simulink model "psm_svpwm_nonlinear_ctrl"  (R2026a)
settings: Solver=ode23tb  StopTime=simlength  FixedStep=tc  MaxStep=tc
values from neighbouring files (symbols this model uses):
  CTRPIFF_CLIP_RELEASE = 0.001    [init_model.m]
  dead_time_INV = 3e-6    (= 3e-06)    [init_model.m]
  emf_fb_p = 0.2    [init_model.m]
  emf_fb_p_ccaller_1 = emf_fb_p    (= 0.2)    [init_model.m]
  emf_fb_p_ccaller_2 = emf_fb_p    (= 0.2)    [init_model.m]
  emf_p = emf_fb_p*4/10    (= 0.08)    [init_model.m]
  emf_p_ccaller_1 = emf_fb_p_ccaller_1*4/10    (= 0.08)    [init_model.m]
  emf_p_ccaller_2 = emf_fb_p_ccaller_2*4/10    (= 0.08)    [init_model.m]
  fPWM_INV = fPWM_AFE    (= 5000)    [init_model.m]
  g0_10Hz = fcut_10Hz_flt * ts_afe * 2*pi    (= 0.0125663706144)    [init_model.m]
  g0_1Hz = fcut_1Hz_flt * ts_afe * 2*pi    (= 0.00125663706144)    [init_model.m]
  g1_10Hz = 1 - g0_10Hz    (= 0.987433629386)    [init_model.m]
  g1_1Hz = 1 - g0_1Hz    (= 0.998743362939)    [init_model.m]
  id_lim = 0.35    [init_model.m]
  inv_m_scale = motorc_m_scale    [init_model.m]
  iq_lim = 1.4    [init_model.m]
  kg = Kobs(1)    [init_model.m]
  ki_align = 0.1    [init_model.m]
  ki_i = 18    [init_model.m]
  ki_w = 8    [init_model.m]
  kp_align = 0.6    [init_model.m]
  kp_i = 0.25    [init_model.m]
  kp_w = 2    [init_model.m]
  kw = Kobs(2)    [init_model.m]
  lim_down_align = -0.2    [init_model.m]
  lim_up_align = 0.2    [init_model.m]
  number_of_modules = 1    [init_model.m]
  omega_m_sim = omega_m_bez    [init_model.m]
  simlength = 2    [init_model.m]
  tc = ts_afe/100    (= 2e-06)    [init_model.m]
  time_gain_afe_module_1 = 1.0    (= 1)    [init_model.m]
  time_gain_inv_module_2 = 1.0    (= 1)    [init_model.m]
  time_start_motor_control = 0.025    [init_model.m]
  ts_inv = 1/fPWM_INV    (= 0.0002)    [init_model.m]
undefined symbols (not defined in the file or in its folder): ibez, La, Lb, Ld_norm, Lq_norm, Ls_norm, magnitude, omega_bez, omega_m_bez, psi_bez, psi_m, psi_m_norm, rpm_base, rpm_bez, Rs, Rs_norm, tau_bez, torque_base, ubez
libraries: fl_lib x24, nesl_utility x11, cstblocks_lti x2, single_phase_pwm_modulator x1, pi_ctrl x1, threephase_inductor_lib x1, simple_flexible_shaft x1, permanent_magnet_synchronous_machine x1
(part 3 of 3)

== system psm_svpwm_nonlinear_ctrl/inv_psm_mod1/inverter_ctrl/inverter_control/current_ctrl/current_ctrl/dq_pi_with_vector_antiwindup mod1/dq_vector_pi ==
  id : Inport
  id_ref : Inport  Port=2
  iq : Inport  Port=3
  iq_ref : Inport  Port=4
  Sum1 : Sum  Inputs=|-+
  Sum2 : Sum  Inputs=|-+
  bounder1 : Subsystem
  bounder2 : Subsystem
  pi_d : Subsystem
  pi_q : Subsystem
  switch : Subsystem
  vector lenght : Subsystem
  md_sat : Outport
  mq_sat : Outport  Port=2
  wires:
  bounder2/2(clip) -> switch/2(clip 2)
  vector lenght/2(m) -> bounder1/3(m), bounder2/1(m)
  Sum2/1 -> pi_q/1(iq_tilde)
  pi_d/1(ud_out) -> vector lenght/1(md), bounder1/1(md)
  pi_q/1(Vqs_out) -> bounder2/3(mq), vector lenght/2(mq)
  vector lenght/1(m_1) -> bounder1/2(m_1), bounder2/2(m_1)
  switch/1(clip) -> pi_q/2(clip), pi_d/2(clip)
  iq/1 -> Sum2/1
  Sum1/1 -> pi_d/1(id_tilde)
  bounder1/2(clip) -> switch/1(clip 1)
  id/1 -> Sum1/1
  bounder1/1(md_sat) -> md_sat/1
  bounder2/1(mq_sat) -> mq_sat/1
  id_ref/1 -> Sum1/2
  iq_ref/1 -> Sum2/2

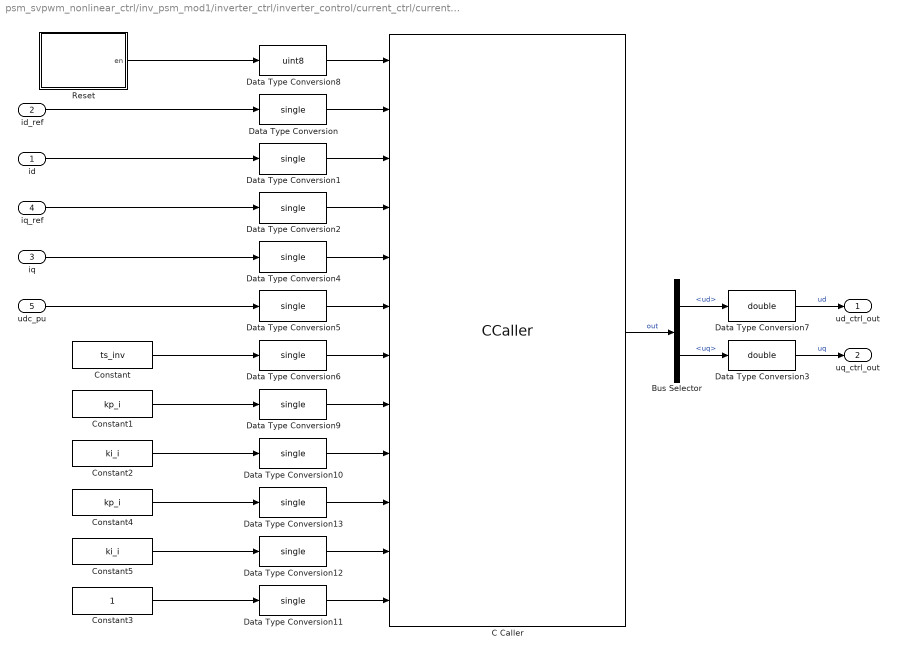
== system psm_svpwm_nonlinear_ctrl/inv_psm_mod1/inverter_ctrl/inverter_control/current_ctrl/current_ctrl/dq_pi_with_vector_antiwindup mod1/dq_vector_pi_ccaller ==
  id : Inport
  id_ref : Inport  Port=2
  iq : Inport  Port=3
  iq_ref : Inport  Port=4
  udc_pu : Inport  Port=5
  Bus Selector : BusSelector  OutputSignals=ud,uq
  C Caller : CCaller  FunctionName=dqvector_pi_process_simulink  PortSpecificationStruct="%)30     .    ,!8   8    (     @         %    \"     T    !     0         %  0 \"0    $    _    07)G3F%M90  4&]R=$YA;64 4V-O<&4     26YD97@     5'EP90      4VEZ90      27-';&]B86P   X    P    !@    @    $          4    (     0    ,    !         !   P!O=70 #@   #     &    \"     0         !0    @    !     P    $         $  # &]U=  .    .     8    (    !          %    \"     $    &     0         0   ...(+7280 chars)"
  Constant : Constant  Value=ts_inv
  Constant1 : Constant  Value=kp_i
  Constant2 : Constant  Value=ki_i
  Constant3 : Constant
  Constant4 : Constant  Value=kp_i
  Constant5 : Constant  Value=ki_i
  Data Type Conversion{,1..2,4..6,9..13} (11 alike) : DataTypeConversion  OutDataTypeStr=single  SaturateOnIntegerOverflow=off  RndMeth=Floor
  Data Type Conversion3 : DataTypeConversion  OutDataTypeStr=double  SaturateOnIntegerOverflow=off  RndMeth=Floor
  Data Type Conversion7 : DataTypeConversion  OutDataTypeStr=double  SaturateOnIntegerOverflow=off  RndMeth=Floor
  Data Type Conversion8 : DataTypeConversion  OutDataTypeStr=uint8  SaturateOnIntegerOverflow=off  RndMeth=Floor
  Reset : Subsystem
  ud_ctrl_out : Outport
  uq_ctrl_out : Outport  Port=2
  wires:
  Data Type Conversion5/1 -> C Caller/6
  Data Type Conversion/1 -> C Caller/2
  C Caller/1 -> Bus Selector/1  "out"
  Data Type Conversion1/1 -> C Caller/3
  Data Type Conversion4/1 -> C Caller/5
  Data Type Conversion2/1 -> C Caller/4
  Data Type Conversion6/1 -> C Caller/7
  Bus Selector/2 -> Data Type Conversion3/1  "<uq>"
  Bus Selector/1 -> Data Type Conversion7/1  "<ud>"
  Data Type Conversion7/1 -> ud_ctrl_out/1  "ud"
  Data Type Conversion3/1 -> uq_ctrl_out/1  "uq"
  Data Type Conversion8/1 -> C Caller/1
  Data Type Conversion9/1 -> C Caller/8
  Data Type Conversion10/1 -> C Caller/9
  Data Type Conversion11/1 -> C Caller/12
  Data Type Conversion13/1 -> C Caller/10
  Data Type Conversion12/1 -> C Caller/11
  Constant3/1 -> Data Type Conversion11/1
  Constant5/1 -> Data Type Conversion12/1
  Constant4/1 -> Data Type Conversion13/1
  Constant2/1 -> Data Type Conversion10/1
  Constant1/1 -> Data Type Conversion9/1
  Constant/1 -> Data Type Conversion6/1
  udc_pu/1 -> Data Type Conversion5/1
  iq/1 -> Data Type Conversion4/1
  iq_ref/1 -> Data Type Conversion2/1
  Reset/1(en) -> Data Type Conversion8/1
  id_ref/1 -> Data Type Conversion/1
  id/1 -> Data Type Conversion1/1

== system psm_svpwm_nonlinear_ctrl/inv_psm_mod1/inverter_ctrl/inverter_control/current_ctrl/bemf_observer/nonlinear_observer/phase_lock_loop/theta_bemf_hat ==
  psi_sd_hat : Inport
  psi_sq_hat : Inport  Port=2
  omega_hat : Inport  Port=3
  Constant1 : Constant  Value=0
  Constant2 : Constant  Value=0
  Gain : Gain  Gain=-1
  Gain1 : Gain  Commented=on  Gain=-1
  Sum : Sum  Inputs=|++
  Trigonometric Function : Trigonometry  Operator=atan2  OutputSignalType=real
  alignment : Scope  NumInputPorts=2
      settings: ActiveDisplayYMinimum=-1.4296113114155271  ActiveDisplayYMaximum=2.2501138881400213  DataLoggingVariableName=ScopeData5
  damped_integral : Subsystem  Commented=on  mask{omega_bez_m=omega_bez, damping_m=0.01, ts_m=ts_inv}
      mask prompts: omega_bez_m "omega_bez"; damping_m "damping"; ts_m "ts"
  damped_integral_with_mod : Subsystem  mask{omega_bez_m=omega_bez, damping_m=0, ts_m=ts_inv}
      mask prompts: omega_bez_m "omega_bez"; damping_m "damping"; ts_m "ts"
  double_integrator_observer : Subsystem  Commented=on
  pi_ctrl : pi_ctrl/pi_ctrl  kp=1  ki=1  ts=ts_inv  lim_up=2  lim_down=-2
  omega_z : Outport  VectorParamsAs1DForOutWhenUnconnected=off
  theta_z : Outport  Port=2  VectorParamsAs1DForOutWhenUnconnected=off
  wires:
  Constant1/1 -> pi_ctrl/1
  Constant2/1 -> pi_ctrl/3
  psi_sq_hat/1 -> Trigonometric Function/1
  Gain1/1 -> double_integrator_observer/1(theta)
  damped_integral_with_mod/1(out) -> theta_z/1
  Sum/1 -> damped_integral_with_mod/1(in), alignment/2, omega_z/1
  psi_sd_hat/1 -> Trigonometric Function/2
  Gain/1 -> pi_ctrl/2
  pi_ctrl/1 -> Sum/1
  omega_hat/1 -> Sum/2
  Trigonometric Function/1 -> Gain/1, alignment/1

== system psm_svpwm_nonlinear_ctrl/inv_psm_mod1/inverter_ctrl/inverter_control/current_ctrl/bemf_observer/nonlinear_observer/psi_dq_hat/psi_d_hat ==
  Gain1 : Gain  Gain=Rs_norm
  Gain3 : Gain  Gain=emf_p
  Gain4 : Gain  Gain=omega_bez
  Gain7 : Gain  Gain=ts_inv
  Product : Product
  Sum : Sum  Inputs=|+-
  Sum2 : Sum  Inputs=++-  SaturateOnIntegerOverflow=on
  Sum3 : Sum  Inputs=|++
  Unit Delay1 : UnitDelay  SampleTime=-1
  tag scope: psi_d_hat_simulink=scoped
  wires:
  Unit Delay1/1 -> Sum3/2, Gain3/1
  Sum2/1 -> Gain4/1
  Gain7/1 -> Sum3/1
  [id_pu_m] -> Gain1/1
  [ud_pu_m] -> Sum/1
  Sum3/1 -> Unit Delay1/1, [psi_d_hat_simulink]
  Gain3/1 -> Sum2/3
  Gain4/1 -> Gain7/1
  Gain1/1 -> Sum/2
  Sum/1 -> Sum2/2
  [omega_z_pu_hat] -> Product/2
  Product/1 -> Sum2/1
  [psi_q_hat_simulink] -> Product/1

== system psm_svpwm_nonlinear_ctrl/inv_psm_mod1/inverter_ctrl/inverter_control/current_ctrl/bemf_observer/nonlinear_observer/psi_dq_hat/psi_q_hat ==
  Gain : Gain  Gain=-1
  Gain1 : Gain  Gain=Rs_norm
  Gain3 : Gain  Gain=emf_p
  Gain4 : Gain  Gain=omega_bez
  Gain7 : Gain  Gain=ts_inv
  Product : Product
  Sum : Sum  Inputs=|+-
  Sum2 : Sum  Inputs=++-  SaturateOnIntegerOverflow=on
  Sum3 : Sum  Inputs=|++
  Unit Delay1 : UnitDelay  SampleTime=-1
  tag scope: psi_q_hat_simulink=scoped
  wires:
  [omega_z_pu_hat] -> Product/2
  Sum/1 -> Sum2/2
  Gain1/1 -> Sum/2
  Gain4/1 -> Gain7/1
  Gain3/1 -> Sum2/3
  Sum3/1 -> [psi_q_hat_simulink], Unit Delay1/1
  [uq_pu_m] -> Sum/1
  [iq_pu_m] -> Gain1/1
  Gain7/1 -> Sum3/1
  Sum2/1 -> Gain4/1
  Unit Delay1/1 -> Sum3/2, Gain3/1
  Product/1 -> Gain/1
  Gain/1 -> Sum2/1
  [psi_d_hat_simulink] -> Product/1

== system psm_svpwm_nonlinear_ctrl/inv_psm_mod1/inverter_ctrl/inverter_control/current_ctrl/current_ctrl/dq_pi_with_vector_antiwindup mod1/dq_vector_pi/bounder1 ==
  md : Inport
  m_1 : Inport  Port=2
  m : Inport  Port=3
  Constant : Constant
  Constant1 : Constant  Value=0
  Divide : Product
  Switch : Switch  Threshold=1  SaturateOnIntegerOverflow=off  InputSameDT=off
  Switch1 : Switch  Threshold=1  SaturateOnIntegerOverflow=off  InputSameDT=off
  md_sat : Outport  VectorParamsAs1DForOutWhenUnconnected=off
  clip : Outport  Port=2  VectorParamsAs1DForOutWhenUnconnected=off
  wires:
  md/1 -> Switch1/3, Divide/2
  m_1/1 -> Divide/1
  Divide/1 -> Switch1/1
  Switch1/1 -> md_sat/1
  Switch/1 -> clip/1
  m/1 -> Switch/2, Switch1/2
  Constant/1 -> Switch/1
  Constant1/1 -> Switch/3

== system psm_svpwm_nonlinear_ctrl/inv_psm_mod1/inverter_ctrl/inverter_control/current_ctrl/current_ctrl/dq_pi_with_vector_antiwindup mod1/dq_vector_pi/bounder2 ==
  m : Inport
  m_1 : Inport  Port=2
  mq : Inport  Port=3
  Constant : Constant
  Constant1 : Constant  Value=0
  Divide : Product
  Switch : Switch  Threshold=1  SaturateOnIntegerOverflow=off  InputSameDT=off
  Switch1 : Switch  Threshold=1  SaturateOnIntegerOverflow=off  InputSameDT=off
  mq_sat : Outport  VectorParamsAs1DForOutWhenUnconnected=off
  clip : Outport  Port=2  VectorParamsAs1DForOutWhenUnconnected=off
  wires:
  Constant1/1 -> Switch/3
  Constant/1 -> Switch/1
  m/1 -> Switch1/2, Switch/2
  Switch/1 -> clip/1
  Switch1/1 -> mq_sat/1
  Divide/1 -> Switch1/1
  m_1/1 -> Divide/1
  mq/1 -> Divide/2, Switch1/3

== system psm_svpwm_nonlinear_ctrl/inv_psm_mod1/inverter_ctrl/inverter_control/current_ctrl/current_ctrl/dq_pi_with_vector_antiwindup mod1/dq_vector_pi/pi_d ==
  id_tilde : Inport
  clip : Inport  Port=2
  1/Ti : Gain  Gain=kp_i  SaturateOnIntegerOverflow=on  OutDataTypeStr=Inherit: Same as input  ParamDataTypeStr=Inherit: Same as input
  Constant : Constant  Value=0
  Sum2 : Sum  Inputs=+-  SaturateOnIntegerOverflow=on
  Sum4 : Sum  SaturateOnIntegerOverflow=on
  Sum5 : Sum  SaturateOnIntegerOverflow=on
  Switch1 : Switch  Threshold=0.5  SaturateOnIntegerOverflow=off  InputSameDT=off
  Switch2 : Switch  Threshold=0.5  SaturateOnIntegerOverflow=off  InputSameDT=off
  Unit Delay1 : UnitDelay  SampleTime=-1
  Unit Delay2 : UnitDelay  SampleTime=-1
  kp1 : Gain  Gain=CTRPIFF_CLIP_RELEASE*ts_inv  SaturateOnIntegerOverflow=on  OutDataTypeStr=Inherit: Same as input  ParamDataTypeStr=Inherit: Same as input
  kp2 : Gain  Gain=ki_i*ts_inv  SaturateOnIntegerOverflow=on  OutDataTypeStr=Inherit: Same as input  ParamDataTypeStr=Inherit: Same as input
  ud_out : Outport  VectorParamsAs1DForOutWhenUnconnected=off
  wires:
  id_tilde/1 -> kp2/1, 1/Ti/1
  Sum5/1 -> ud_out/1
  Switch1/1 -> Unit Delay2/1
  Sum4/1 -> Sum5/2, Switch1/3
  kp1/1 -> Sum2/2
  Sum2/1 -> Switch1/1
  Unit Delay2/1 -> Sum4/2, kp1/1, Sum2/1
  1/Ti/1 -> Sum5/1
  Switch2/1 -> Sum4/1
  kp2/1 -> Switch2/3
  clip/1 -> Unit Delay1/1
  [clip] -> Switch2/2
  [clip] -> Switch1/2
  Constant/1 -> Switch2/1
  Unit Delay1/1 -> [clip]

== system psm_svpwm_nonlinear_ctrl/inv_psm_mod1/inverter_ctrl/inverter_control/current_ctrl/current_ctrl/dq_pi_with_vector_antiwindup mod1/dq_vector_pi/pi_q ==
  iq_tilde : Inport
  clip : Inport  Port=2
  1/Ti : Gain  Gain=kp_i  SaturateOnIntegerOverflow=on  OutDataTypeStr=Inherit: Same as input  ParamDataTypeStr=Inherit: Same as input
  Constant : Constant  Value=0
  Sum2 : Sum  Inputs=+-  SaturateOnIntegerOverflow=on
  Sum4 : Sum  SaturateOnIntegerOverflow=on
  Sum5 : Sum  SaturateOnIntegerOverflow=on
  Switch1 : Switch  Threshold=0.5  SaturateOnIntegerOverflow=off  InputSameDT=off
  Switch2 : Switch  Threshold=0.5  SaturateOnIntegerOverflow=off  InputSameDT=off
  Unit Delay1 : UnitDelay  SampleTime=-1
  Unit Delay2 : UnitDelay  SampleTime=-1
  kp1 : Gain  Gain=CTRPIFF_CLIP_RELEASE*ts_inv  SaturateOnIntegerOverflow=on  OutDataTypeStr=Inherit: Same as input  ParamDataTypeStr=Inherit: Same as input
  kp2 : Gain  Gain=ki_i*ts_inv  SaturateOnIntegerOverflow=on  OutDataTypeStr=Inherit: Same as input  ParamDataTypeStr=Inherit: Same as input
  Vqs_out : Outport  VectorParamsAs1DForOutWhenUnconnected=off
  wires:
  Constant/1 -> Switch2/1
  [clip] -> Switch1/2
  [clip] -> Switch2/2
  clip/1 -> Unit Delay1/1
  kp2/1 -> Switch2/3
  Switch2/1 -> Sum4/1
  1/Ti/1 -> Sum5/1
  Unit Delay2/1 -> Sum2/1, kp1/1, Sum4/2
  Sum2/1 -> Switch1/1
  kp1/1 -> Sum2/2
  Sum4/1 -> Sum5/2, Switch1/3
  Switch1/1 -> Unit Delay2/1
  iq_tilde/1 -> 1/Ti/1, kp2/1
  Unit Delay1/1 -> [clip]
  Sum5/1 -> Vqs_out/1

== system psm_svpwm_nonlinear_ctrl/inv_psm_mod1/inverter_ctrl/inverter_control/current_ctrl/current_ctrl/dq_pi_with_vector_antiwindup mod1/dq_vector_pi/switch ==
  clip 1 : Inport
  clip 2 : Inport  Port=2
  Constant4 : Constant
  Constant5 : Constant  Value=0
  Sum1 : Sum  SaturateOnIntegerOverflow=on
  Switch : Switch  Threshold=0.5  SaturateOnIntegerOverflow=off  InputSameDT=off
  clip : Outport  VectorParamsAs1DForOutWhenUnconnected=off
  wires:
  Constant5/1 -> Switch/3
  Switch/1 -> clip/1
  Constant4/1 -> Switch/1
  Sum1/1 -> Switch/2
  clip 1/1 -> Sum1/1
  clip 2/1 -> Sum1/2

== system psm_svpwm_nonlinear_ctrl/inv_psm_mod1/inverter_ctrl/inverter_control/current_ctrl/current_ctrl/dq_pi_with_vector_antiwindup mod1/dq_vector_pi/vector lenght ==
  md : Inport
  mq : Inport  Port=2
  Math Function : Math  Operator=magnitude^2  SignedPower=on
  Math Function1 : Math  Operator=magnitude^2  SignedPower=on
  Math Function2 : Math  Operator=reciprocal  SignedPower=on
  Sqrt : Sqrt
  Sum5 : Sum  SaturateOnIntegerOverflow=on
  m_1 : Outport  VectorParamsAs1DForOutWhenUnconnected=off
  m : Outport  Port=2  VectorParamsAs1DForOutWhenUnconnected=off
  wires:
  Sqrt/1 -> m/1, Math Function2/1
  mq/1 -> Math Function1/1
  Math Function1/1 -> Sum5/2
  Math Function/1 -> Sum5/1
  Sum5/1 -> Sqrt/1
  Math Function2/1 -> m_1/1
  md/1 -> Math Function/1

== system psm_svpwm_nonlinear_ctrl/inv_psm_mod1/inverter_ctrl/inverter_control/current_ctrl/current_ctrl/dq_pi_with_vector_antiwindup mod1/dq_vector_pi_ccaller/Reset ==
  Step : Step  Time=0.05  InitialValue=1  FinalValue=0
  en : Outport
  wires:
  Step/1 -> en/1

== system psm_svpwm_nonlinear_ctrl/inv_psm_mod1/inverter_ctrl/inverter_control/current_ctrl/bemf_observer/nonlinear_observer/phase_lock_loop/theta_bemf_hat/damped_integral ==
  in : Inport
  Gain3 : Gain  Gain=damping_m
  Gain4 : Gain  Gain=omega_bez_m
  Gain7 : Gain  Gain=ts_m
  Sum2 : Sum  Inputs=+-  SaturateOnIntegerOverflow=on
  Sum3 : Sum  Inputs=|++
  Unit Delay1 : UnitDelay  SampleTime=-1
  out : Outport
  wires:
  Sum2/1 -> Gain4/1
  Gain7/1 -> Sum3/1
  Sum3/1 -> Unit Delay1/1
  Unit Delay1/1 -> Gain3/1, Sum3/2, out/1
  Gain4/1 -> Gain7/1
  in/1 -> Sum2/1
  Gain3/1 -> Sum2/2

== system psm_svpwm_nonlinear_ctrl/inv_psm_mod1/inverter_ctrl/inverter_control/current_ctrl/bemf_observer/nonlinear_observer/phase_lock_loop/theta_bemf_hat/damped_integral_with_mod ==
  in : Inport
  Gain3 : Gain  Gain=damping_m
  Gain4 : Gain  Gain=omega_bez_m
  Gain7 : Gain  Gain=ts_m
  Sum2 : Sum  Inputs=+-  SaturateOnIntegerOverflow=on
  Sum3 : Sum  Inputs=|++
  Unit Delay1 : UnitDelay  SampleTime=-1
  bounder1 : MATLAB Function  TreatAsAtomicUnit=on
  out : Outport
  wires:
  Gain3/1 -> Sum2/2
  in/1 -> Sum2/1
  Gain4/1 -> Gain7/1
  Unit Delay1/1 -> bounder1/1(u)
  Sum3/1 -> Unit Delay1/1
  Gain7/1 -> Sum3/1
  Sum2/1 -> Gain4/1
  bounder1/1(y) -> out/1, Sum3/2, Gain3/1

== system psm_svpwm_nonlinear_ctrl/inv_psm_mod1/inverter_ctrl/inverter_control/current_ctrl/bemf_observer/nonlinear_observer/phase_lock_loop/theta_bemf_hat/double_integrator_observer ==
  theta : Inport
  Gain : Gain  Gain=kw
  Gain1 : Gain  Gain=kg
  Gain2 : Gain  Gain=omega_bez
  Gain3 : Gain  Gain=1/omega_bez
  Gain5 : Gain  Gain=ts_inv
  Sum : Sum  Inputs=-+|
  Sum1 : Sum  Inputs=|++
  Sum2 : Sum  Inputs=|++
  Sum8 : Sum  Inputs=++|
  Unit Delay1 : UnitDelay  InitialCondition=pi  SampleTime=-1
  Unit Delay2 : UnitDelay  SampleTime=-1
  bounder1 : MATLAB Function  TreatAsAtomicUnit=on
  bounder2 : MATLAB Function  TreatAsAtomicUnit=on
  omega_z_pu_hat : Outport  VectorParamsAs1DForOutWhenUnconnected=off
  theta_z_hat : Outport  Port=2  VectorParamsAs1DForOutWhenUnconnected=off
  wires:
  Gain1/1 -> Sum2/1
  theta/1 -> Sum/2  "theta_bemf"
  Sum8/1 -> Unit Delay1/1
  Unit Delay1/1 -> bounder2/1(u)
  Sum1/1 -> Unit Delay2/1
  Gain/1 -> Gain3/1
  Unit Delay2/1 -> omega_z_pu_hat/1, Sum1/2, Gain5/1
  Sum2/1 -> Sum8/2
  bounder2/1(y) -> Sum2/2, theta_z_hat/1, Sum/1
  bounder1/1(y) -> Gain1/1, Gain/1
  Gain2/1 -> Sum8/1
  Gain3/1 -> Sum1/1
  Gain5/1 -> Gain2/1
  Sum/1 -> bounder1/1(u)

== matlab function psm_svpwm_nonlinear_ctrl/inv_psm_mod1/inverter_ctrl/inverter_control/current_ctrl/current_transformation/alphabeta2dq ==
  data: alpha input; d output; beta input; gamma input; q output
function [d,q] = alphabeta2dq(alpha,beta,gamma)

    d  =  alpha*cos(gamma) + beta*sin(gamma);
    q = -alpha*sin(gamma) + beta*cos(gamma);

end

== matlab function psm_svpwm_nonlinear_ctrl/inv_psm_mod1/inverter_ctrl/inverter_control/current_ctrl/bemf_observer/nonlinear_observer/phase_lock_loop/theta_bemf_hat/double_integrator_observer/bounder1 ==
  data: u input; y output
function y = bounder(u)
    
    y = -pi + mod(u+3*pi,2*pi);
end

== matlab function psm_svpwm_nonlinear_ctrl/inv_psm_mod1/inverter_ctrl/inverter_control/current_ctrl/bemf_observer/nonlinear_observer/phase_lock_loop/theta_bemf_hat/double_integrator_observer/bounder2 ==
  data: u input; y output
function y = bounder(u)
    
    u = -pi + mod(u+3*pi,2*pi);
    
    y = u;
end

== matlab function psm_svpwm_nonlinear_ctrl/inv_psm_mod1/inverter_ctrl/inverter_control/current_ctrl/bemf_observer/nonlinear_observer/phase_lock_loop/alphabeta2dq ==
  data: alpha input; d output; beta input; gamma input; q output
function [d,q] = alphabeta2dq(alpha,beta,gamma)

    d  =  alpha*cos(gamma) + beta*sin(gamma);
    q = -alpha*sin(gamma) + beta*cos(gamma);

end

== matlab function psm_svpwm_nonlinear_ctrl/inv_psm_mod1/inverter_ctrl/inverter_control/current_ctrl/current_transformation/uvw2alphabeta ==
  data: u input; alpha output; v input; w input; beta output
function [alpha,beta] = uvw2alphabeta(u,v,w)

alpha = 2/3*(u - 1/2*v - 1/2*w);
beta  = 2/3*(sqrt(3)/2*(v - w));

end

== matlab function psm_svpwm_nonlinear_ctrl/inv_psm_mod1/inverter_ctrl/inverter_control/current_ctrl/current_ctrl/output voltage transformation/dq2alphabeta ==
  data: d input; alpha output; q input; gamma input; beta output
function [alpha,beta] = dq2alphabeta(d,q,gamma)

    alpha  =  d*cos(gamma) - q*sin(gamma);
    beta = d*sin(gamma) + q*cos(gamma);

end

== matlab function psm_svpwm_nonlinear_ctrl/inv_psm_mod1/inverter_ctrl/inverter_control/current_ctrl/bemf_observer/bemf_observer/double_integrator_observer/bounder1 ==
  data: u input; y output
function y = bounder(u)
    
    y = -pi + mod(u+3*pi,2*pi);
end

== matlab function psm_svpwm_nonlinear_ctrl/inv_psm_mod1/inverter_ctrl/inverter_control/current_ctrl/bemf_observer/bemf_observer/double_integrator_observer/bounder2 ==
  data: u input; y output
function y = bounder(u)
    
    u = -pi + mod(u+3*pi,2*pi);
    
    y = u;
end

== matlab function psm_svpwm_nonlinear_ctrl/inv_psm_mod1/inverter/timer/MATLAB Function ==
  data: t input; y output; phase input; period input
function y = ramp_up_down(t,phase,period)
x = sin(2*pi/period*t - phase -pi/2);
y = asin(x)/pi + 1/2;

== matlab function psm_svpwm_nonlinear_ctrl/inv_psm_mod1/inverter_ctrl/inverter_control/encoder-sensorless-switch/double_integrator_observer/bounder1 ==
  data: u input; y output
function y = bounder(u)
    y = -pi + mod(u+3*pi,2*pi);
end

== matlab function psm_svpwm_nonlinear_ctrl/inv_psm_mod1/inverter_ctrl/inverter_control/encoder-sensorless-switch/double_integrator_observer/bounder2 ==
  data: u input; y output
function y = bounder(u)
    y = -pi + mod(u+3*pi,2*pi);
end

== matlab function psm_svpwm_nonlinear_ctrl/inv_psm_mod1/inverter_ctrl/inverter_control/current_ctrl/bemf_observer/nonlinear_observer/phase_lock_loop/theta_bemf_hat/damped_integral_with_mod/bounder1 ==
  data: u input; y output
function y = bounder(u)
    
    y = -pi + mod(u+3*pi,2*pi);
end

== matlab function psm_svpwm_nonlinear_ctrl/inv_psm_mod1/inverter/MATLAB Function ==
  data: ua input; uu output; uv output; uw output; ub input
function [uu, uv, uw] = ab2uvw(ua, ub)

uu = ua;
uv = -ua/2 + sqrt(3)/2*ub;
uw = -ua/2 - sqrt(3)/2*ub;

== matlab function psm_svpwm_nonlinear_ctrl/inv_psm_mod1/inverter_ctrl/inverter_control/encoder-sensorless-switch/MATLAB Function ==
  data: omega_ctrl output; phase_psm input; omega_obs input; phase_obs input; phase_ctrl output; omega_psm input; omega_th parameter
function [omega_ctrl, phase_ctrl] = switch_enc2obs(phase_psm, omega_obs, phase_obs, omega_psm, omega_th)

if abs(omega_psm) > omega_th
    omega_ctrl = omega_obs;
    phase_ctrl = phase_obs;
else
    omega_ctrl = omega_psm;
    phase_ctrl = phase_psm;
end

== matlab function psm_svpwm_nonlinear_ctrl/inv_psm_mod1/inverter_ctrl/inverter_control/current_ctrl/bemf_observer/nonlinear_observer/MATLAB Function ==
  data: i_sd input; isd_h_new output; i_sq input; u_sd input; u_sq input; omega_0 input; i_sd_ref input; i_sq_ref input; isd_h input; isq_h input; psi_sd_h input; psi_sq_h input; chi_d_h input; chi_q_h input; omega_h input; Ls input; Rs input; gamma input; kp input; ki input; k_psi input; phi_m input; ts input; isq_h_new output; psi_sd_h_new output; psi_sq_h_new output; chi_d_h_new output; chi_q_h_new output; omega_h_new output; eta_d output; eta_q output; xi_sd output; xi_sq output; omega_bez input; emf_p input
function [isd_h_new, isq_h_new, psi_sd_h_new, psi_sq_h_new, ...
          chi_d_h_new, chi_q_h_new, omega_h_new, ...
          eta_d, eta_q, xi_sd, xi_sq] = ...
    nlobs(i_sd, i_sq, u_sd, u_sq, omega_0, ...
          i_sd_ref, i_sq_ref, ...
          isd_h, isq_h, psi_sd_h, psi_sq_h, ...
          chi_d_h, chi_q_h, omega_h, ...
          Ls, Rs, gamma, kp, ki, k_psi, phi_m, ts, omega_bez, emf_p)
% NLOBS  Nonlinear observer - discrete-time MATLAB Function block
%        Stati x[k-1] in ingresso, stati x[k] in uscita (z^-1 esterni)
%
% Discretizzazione: Eulero in avanti (Forward Euler)
%
% Ingressi:
%   i_sd, i_sq       : correnti statoriali misurate [A] (frame dq)
%   u_sd, u_sq       : tensioni statoriali [V]
%   omega_0          : pulsazione sincrona [rad/s]
%   i_sd_ref, i_sq_ref : riferimenti di corrente
%   isd_h, isq_h     : stima correnti (stato k-1)
%   psi_sd_h, psi_sq_h : stima flussi (stato k-1)
%   chi_d_h, chi_q_h : stati integratori (stato k-1)
%   omega_h          : stima velocita' (stato k-1)
%   Ls, Rs           : induttanza e resistenza statoriale
%   p                : numero coppie polari
%   gamma            : guadagno adattivo velocita'
%   kp, ki           : guadagni proporzionale/integrale corrente
%   k_psi            : guadagno flusso
%   phi_m            : flusso magnete permanente [Wb]
%   ts               : periodo di campionamento [s]

%--- Errori di corrente (tilde)
i_tilde_sd = i_sd - isd_h;
i_tilde_sq = i_sq - isq_h;

%--- Termini di iniezione corrente
eta_d =  kp * i_tilde_sd + chi_q_h;
eta_q =  kp * i_tilde_sq - chi_d_h;

%--- Flussi di riferimento
psi_sd_ref = phi_m + Ls * i_sd_ref;
psi_sq_ref =         Ls * i_sq_ref;

%--- Termini di iniezione flusso
xi_sd = -k_psi * (psi_sd_h - psi_sd_ref);
xi_sq = -k_psi * (psi_sq_h - psi_sq_ref);

%--- Flussi di rotore stimati (lambda_r = psi_s - Ls*is)
lambda_sd = psi_sd_h - Ls * isd_h;   % psi_sq - Ls*isq lato q
lambda_sq = psi_sq_h - Ls * isq_h;

%--- Derivate degli stati (equazioni continue) --------------------

% d/dt isd_hat
d_isd_h = (1/Ls) * ( -Rs*isd_h ...
                     + (omega_0 - omega_h)*Ls*i_sq ...
                     + omega_h*psi_sq_h ...
                     + u_sd + eta_d );

% d/dt isq_hat
d_isq_h = (1/Ls) * ( -Rs*isq_h ...
                     - (omega_0 - omega_h)*Ls*i_sd ...
                     - omega_h*psi_sd_h ...
                     + u_sq + eta_q );

% d/dt psi_sd_hat
d_psi_sd = -Rs*i_sd + omega_0*psi_sq_h + u_sd + xi_sd - emf_p*psi_sd_h;

% d/dt psi_sq_hat
d_psi_sq = -Rs*i_sq - omega_0*psi_sd_h + u_sq + xi_sq - emf_p*psi_sq_h;

% d/dt chi_d
d_chi_d =  omega_0*chi_q_h - ki*i_tilde_sq;

% d/dt chi_q
d_chi_q = -omega_0*chi_d_h + ki*i_tilde_sd;

% d/dt omega_hat
d_omega = (1/gamma) * ( lambda_sq*i_tilde_sd - lambda_sd*i_tilde_sq );

%--- Integrazione Forward Euler -----------------------------------
isd_h_new   = isd_h   + ts * omega_bez * d_isd_h;
isq_h_new   = isq_h   + ts * omega_bez * d_isq_h;
psi_sd_h_new = psi_sd_h + ts * omega_bez * d_psi_sd;
psi_sq_h_new = psi_sq_h + ts * omega_bez * d_psi_sq;
chi_d_h_new  = chi_d_h  + ts * omega_bez * d_chi_d;
chi_q_h_new  = chi_q_h  + ts * omega_bez * d_chi_q;
omega_h_new  = omega_h  + ts * omega_bez * d_omega;

end
